simulink model "double_integrator"  (R2018b)
settings: Solver=FixedStepDiscrete  StartTime=0.0  StopTime=length(noise_y)*dt  FixedStep=dt  RelTol=1e-3
values from neighbouring files (symbols this model uses):
  dt = 1    [get_parameters.m]
  sysd = c2d(sys, dt)    [get_parameters.m]
undefined symbols (not defined in the file or in its folder): Kd
libraries: simulink x2
settings Model: Creator=cornell  LastModifiedBy=cornell
settings DataIOCC: SaveOutput=off  SignalLogging=off  DSMLogging=off  SaveTime=off

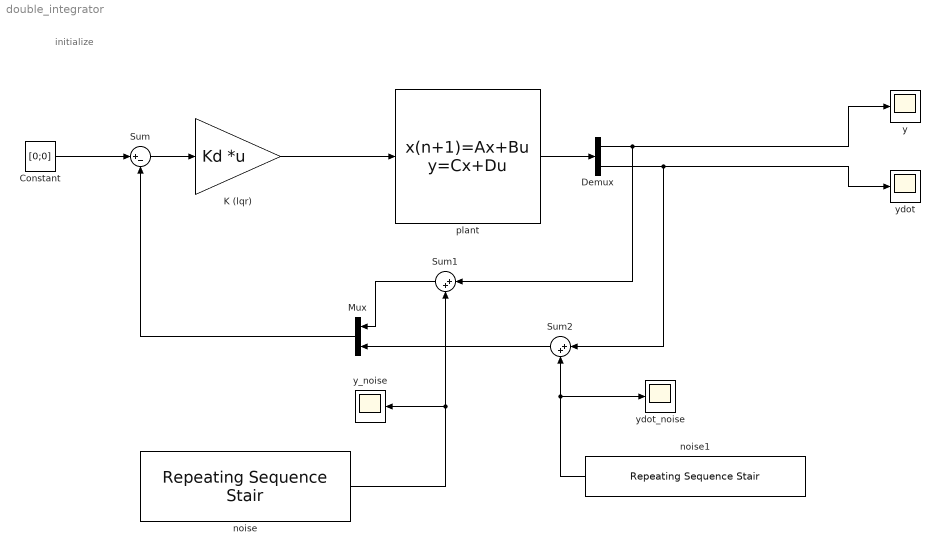
== system double_integrator ==
  note: initialize
  Constant : Constant  Value=[0;0]  SampleTime=1
  Demux : Demux  Outputs=2
  K (lqr) : Gain  Gain=Kd  Multiplication=Matrix(K*u) (u vector)
  Mux : Mux  Inputs=2
  Sum : Sum  Inputs=|+-
  Sum1 : Sum  Inputs=|++
  Sum2 : Sum  Inputs=|++
  noise : simulink/Sources/Repeating Sequence Stair  OutValues=noise_y  tsamp=1  OutMin=[]  OutMax=[]  OutDataTypeStr=double  OutputDataTypeScalingMode=double  OutDataType=fixdt(0,8)  ConRadixGroup=Best Precision: Vector-wise  OutScaling=2^-12
  noise1 : simulink/Sources/Repeating Sequence Stair  OutValues=noise_ydot  tsamp=1  OutMin=[]  OutMax=[]  OutDataTypeStr=double  OutputDataTypeScalingMode=double  OutDataType=fixdt(0,8)  ConRadixGroup=Best Precision: Vector-wise  OutScaling=2^-12
  plant : DiscreteStateSpace  A=sysd.A  B=sysd.B  C=sysd.C  D=sysd.D  InitialCondition=[0;0]  SampleTime=dt
  y : Scope
  y_noise : Scope
  ydot : Scope
  ydot_noise : Scope
  wires:
  plant/1 -> Demux/1
  K (lqr)/1 -> plant/1
  Sum/1 -> K (lqr)/1
  Constant/1 -> Sum/1
  Demux/1 -> Sum1/1, y/1
  Demux/2 -> Sum2/1, ydot/1
  Sum1/1 -> Mux/1
  noise/1 -> y_noise/1, Sum1/2
  Mux/1 -> Sum/2
  Sum2/1 -> Mux/2
  noise1/1 -> ydot_noise/1, Sum2/2
